simulink model "Main_model"  (R2021b)
settings: Solver=ode23t  StartTime=0.0  StopTime=sim_t_end  RelTol=1e-3
undefined symbols (not defined in the file): ambient_co2, ambient_pressure, ambient_rh, ambient_temp, battery, battery_heat_gen_scale, battery_mass, battery_thermal_mass, cab_air_v_dot, cabin_heater_cmd, cabin_heater_max_power, case_cold_plate_mass, case_cold_plate_thermal_mass, chiller_baffles_n, chiller_tube_length, chiller_tubes_n_rows, compressor_max_m_dot, compressor_ref_m_dot, condenser_air_min_flow_area, condenser_tube_width, const_current, coolant_channel_length, coolant_initial_T, coolant_m_dot, coolant_pipe_cross_sec_area, evaporator_air_cross_sec_area, evaporator_air_min_flow_area, evaporator_tube_width, motor_mc_heat_fraction, n_parallel, power_fraction_rear, ptc_heater_max_power, ptc_heater_thermal_mass, rad_air_v_dot, radiator_air_cross_sec_area, radiator_air_min_flow_area, radiator_tube_width, ref_m_dot, ref_pipe_dia, refrigerant_initial_void_fraction, refrigerant_pipe_cross_sec_area, T_bat_active_cool, T_bat_active_heat, T_bat_passive_cool, T_bat_passive_heat, T_battery_init, T_battery_nom, T_cabin_init, T_cabin_setpoint, T_dcdc_nom, T_DT_high, T_DT_passive_cool, T_DT_whr_active, T_front_gb_nom, T_front_mc_nom, T_front_motor_nom, T_rear_gb_nom, T_rear_mc_nom, T_rear_motor_nom, three_w_valve_max_open_area_factor ... (+3)
libraries: fl_lib x448, nesl_utility x328, SimscapeFluids_lib x134, slpidlib x15, ee_lib x9, simulink x8, LiBatteryElements_lib x4, SignalEditorBlockLib x1
(part 2 of 24)

== system Main_model/Compressor ==
  Absolute Reference (2P) : fl_lib/Two-Phase Fluid/Elements/Absolute Reference (2P)
      settings: SourceProductBaseCode=SS
  Absolute Reference (2P)1 : fl_lib/Two-Phase Fluid/Elements/Absolute Reference (2P)
      settings: SourceProductBaseCode=SS
  Constant1 : Constant  Value=1/.7-1
  Constant2 : Constant
  PS-Simulink Converter1 : nesl_utility/PS-Simulink Converter  PhysicalDomain=network_engine_domain  SubClassName=ps_output  LeftPortType=input  RightPortType=output  PseudoPeriodic=off  Frequencies=[]  Unit=MPa  AffineConversion=off
      settings: SourceProductBaseCode=PW,SS
  PS-Simulink Converter2 : nesl_utility/PS-Simulink Converter  PhysicalDomain=network_engine_domain  SubClassName=ps_output  LeftPortType=input  RightPortType=output  PseudoPeriodic=off  Frequencies=[]  Unit=MPa  AffineConversion=off
      settings: SourceProductBaseCode=PW,SS
  PS-Simulink Converter3 : nesl_utility/PS-Simulink Converter  PhysicalDomain=network_engine_domain  SubClassName=ps_output  LeftPortType=input  RightPortType=output  PseudoPeriodic=off  Frequencies=[]  Unit=K  AffineConversion=off
      settings: SourceProductBaseCode=PW,SS
  PS-Simulink Converter4 : nesl_utility/PS-Simulink Converter  PhysicalDomain=network_engine_domain  SubClassName=ps_output  LeftPortType=input  RightPortType=output  PseudoPeriodic=off  Frequencies=[]  Unit=K  AffineConversion=off
      settings: SourceProductBaseCode=PW,SS
  PS-Simulink Converter5 : nesl_utility/PS-Simulink Converter  PhysicalDomain=network_engine_domain  SubClassName=ps_output  LeftPortType=input  RightPortType=output  PseudoPeriodic=off  Frequencies=[]  Unit=1  AffineConversion=off
      settings: SourceProductBaseCode=PW,SS
  PS-Simulink Converter6 : nesl_utility/PS-Simulink Converter  PhysicalDomain=network_engine_domain  SubClassName=ps_output  LeftPortType=input  RightPortType=output  PseudoPeriodic=off  Frequencies=[]  Unit=1  AffineConversion=off
      settings: SourceProductBaseCode=PW,SS
  Pressure & Internal Energy Sensor (2P) : fl_lib/Two-Phase Fluid/Sensors/Pressure & Internal Energy Sensor (2P)
      settings: SourceProductBaseCode=SS  InternalSimscapePortConfiguration="{\"Bottom\":[],\"Left\":[{\"id\":\"A\",\"label\":\"A\",\"type\":\"foundation.two_phase_fluid.two_phase_fluid\"}],\"Right\":[{\"id\":\"B\",\"label\":\"B\",\"type\":\"foundation.two_phase_fluid.two_phase_fluid\"},{\"id\":\"P\",\"label\":\"P\",\"type\":\"output\"},{\"id\":\"U\",\"label\":\"U\",\"type\":\"output\"}],\"Top\":[]}"
  Pressure & Internal Energy Sensor (2P)1 : fl_lib/Two-Phase Fluid/Sensors/Pressure & Internal Energy Sensor (2P)
      settings: SourceProductBaseCode=SS  InternalSimscapePortConfiguration="{\"Bottom\":[],\"Left\":[{\"id\":\"A\",\"label\":\"A\",\"type\":\"foundation.two_phase_fluid.two_phase_fluid\"}],\"Right\":[{\"id\":\"B\",\"label\":\"B\",\"type\":\"foundation.two_phase_fluid.two_phase_fluid\"},{\"id\":\"P\",\"label\":\"P\",\"type\":\"output\"},{\"id\":\"U\",\"label\":\"U\",\"type\":\"output\"}],\"Top\":[]}"
  R1234yf Properties : SimscapeFluids_lib/Two-Phase Fluid/Utilities/Two-Phase Fluid Predefined Properties (2P)  fluid=fluids.two_phase_fluid.utilities.enum.Fluid.R1234yf  p_atm=ambient_pressure MPa  q_rev=0.01 Pa
      settings: SourceProductBaseCode=SH
  "Refrigerant Mass Flow Rate Controls " : Subsystem
  Scope : Scope
  Simulink-PS Converter1 : nesl_utility/Simulink-PS Converter  PhysicalDomain=network_engine_domain  SubClassName=ps_input  LeftPortType=input  RightPortType=output  PseudoPeriodic=off  Frequencies=[]  NoiseDistribution=none  NoiseParameters=[]  Unit=1  AffineConversion=off  FilteringAndDerivatives=provide  SimscapeFilterOrder=1  InputFilterTimeConstant=0.001  UdotUserProvided=0
      settings: SourceProductBaseCode=PW,SS
  Sum : Sum  Inputs=|++
  Thermodynamic Properties Sensor (2P) : fl_lib/Two-Phase Fluid/Sensors/Thermodynamic Properties Sensor (2P)
      settings: SourceProductBaseCode=SS  InternalSimscapePortConfiguration="{\"Bottom\":[],\"Left\":[{\"id\":\"A\",\"label\":\"A\",\"type\":\"foundation.two_phase_fluid.two_phase_fluid\"}],\"Right\":[{\"id\":\"T\",\"label\":\"T\",\"type\":\"output\"},{\"id\":\"H\",\"label\":\"h\",\"type\":\"output\"},{\"id\":\"V\",\"label\":\"v\",\"type\":\"output\"},{\"id\":\"S\",\"label\":\"s\",\"type\":\"output\"}],\"Top\":[]}"
  Thermodynamic Properties Sensor (2P)1 : fl_lib/Two-Phase Fluid/Sensors/Thermodynamic Properties Sensor (2P)
      settings: SourceProductBaseCode=SS  InternalSimscapePortConfiguration="{\"Bottom\":[],\"Left\":[{\"id\":\"A\",\"label\":\"A\",\"type\":\"foundation.two_phase_fluid.two_phase_fluid\"}],\"Right\":[{\"id\":\"T\",\"label\":\"T\",\"type\":\"output\"},{\"id\":\"H\",\"label\":\"h\",\"type\":\"output\"},{\"id\":\"V\",\"label\":\"v\",\"type\":\"output\"},{\"id\":\"S\",\"label\":\"s\",\"type\":\"output\"}],\"Top\":[]}"
  Transfer Fcn : TransferFcn  Denominator=[100 1]
  compressor : SimscapeComponentBlock  SourceFile=custom.self_controlled_mass_flow_source  ComponentPath=custom.self_controlled_mass_flow_source  ComponentVariants="[\"custom.self_controlled_mass_flow_source\"]"  ComponentVariantNames="[\"self_controlled_mass_flow_source\"]"  ClassName=self_controlled_mass_flow_source  SchemaVersion=1  power_spec=foundation.enum.power_spec.isentropic  area_A=refrigerant_pipe_cross_sec_area m^2  area_B=refrigerant_pipe_cross_sec_area m^2
      settings: CopyFcn=simscape.engine.sli.internal.componentblockcallback(gcbh,'COPY')  PreCopyFcn=simscape.engine.sli.internal.componentblockcallback(gcbh,'PRECOPY')  PreDeleteFcn=simscape.engine.sli.internal.componentblockcallback(gcbh,'PREDELETE')  InternalSimscapePortConfiguration="{\"Bottom\":[],\"Left\":[{\"id\":\"A\",\"label\":\"A\",\"type\":\"foundation.two_phase_fluid.two_phase_fluid\"},{\"id\":\"M\",\"label\":\"M\",\"type\":\"input\"},{\"id\":\"eff\",\"label\":\"eff\",\"type\":\"input\"}],\"Right\":[{\"id\":\"B\",\"label\":\"B\",\"type\":\"foundation.two_phase_fluid.two_phase_fluid\"}],\"Top\":[]}"
      mask Type: Controlled Mass Flow Rate Source (2P)
  heat loss : Subsystem
  Ref Out : PMIOPort  Side=Left
  Ref in : PMIOPort  Port=2  Side=Right
  tag scope: T_cond_comp_in=global, T_evap_comp_in=global, h_cond_comp_in=global, h_evap_comp_in=global, p_cond_comp_in=global, p_evap_comp_in=global
  wires:
  PS-Simulink Converter1/1 -> [p_evap_comp_in]
  PS-Simulink Converter2/1 -> [p_cond_comp_in]
  Sum/1 -> Scope/1, Simulink-PS Converter1/1
  Constant1/1 -> Transfer Fcn/1
  Constant2/1 -> Sum/2
  Transfer Fcn/1 -> Sum/1
  PS-Simulink Converter3/1 -> [T_evap_comp_in]
  PS-Simulink Converter5/1 -> [h_evap_comp_in]
  PS-Simulink Converter6/1 -> [h_cond_comp_in]
  PS-Simulink Converter4/1 -> [T_cond_comp_in]
  connections:
  PS-Simulink Converter1/LConn1 -- Pressure & Internal Energy Sensor (2P)/RConn2
  Pressure & Internal Energy Sensor (2P)/RConn1 -- Absolute Reference (2P)/LConn1
  Pressure & Internal Energy Sensor (2P)1/RConn1 -- Absolute Reference (2P)1/LConn1
  PS-Simulink Converter2/LConn1 -- Pressure & Internal Energy Sensor (2P)1/RConn2
  Pressure & Internal Energy Sensor (2P)1/LConn1 -- heat loss/LConn1 -- compressor/RConn1 -- Thermodynamic Properties Sensor (2P)1/LConn1
  heat loss/RConn1 -- Ref Out/RConn1
  "Refrigerant Mass Flow Rate Controls "/RConn1 -- compressor/LConn2
  compressor/LConn1 -- Pressure & Internal Energy Sensor (2P)/LConn1 -- R1234yf Properties/RConn1 -- Ref in/RConn1 -- Thermodynamic Properties Sensor (2P)/LConn1
  Simulink-PS Converter1/RConn1 -- compressor/LConn3
  Thermodynamic Properties Sensor (2P)/RConn2 -- PS-Simulink Converter5/LConn1
  PS-Simulink Converter3/LConn1 -- Thermodynamic Properties Sensor (2P)/RConn1
  Thermodynamic Properties Sensor (2P)1/RConn2 -- PS-Simulink Converter6/LConn1
  Thermodynamic Properties Sensor (2P)1/RConn1 -- PS-Simulink Converter4/LConn1

== system Main_model/Condenser ==
  Pump : Subsystem
  condenser : Subsystem
      settings: PortSchema="{\"entries\":[{\"content\":{\"sides\":[{\"content\":{\"connectorIds\":[]},\"type\":\"ConnectorPlacement.EquallySpacedRectSide\",\"uuid\":\"3be5e3bd-c423-4591-b0f7-380c1ba81e55\"},{\"content\":{\"connectorIds\":[],\"side\":\"RIGHT\"},\"type\":\"ConnectorPlacement.EquallySpacedRectSide\",\"uuid\":\"149d4538-0447-4c3c-bea8-6305fc9625c0\"},{\"content\":{\"connectorIds\":[\"LConn1\",\"LConn2\"],\"side\":\"TOP\"},\"type\":\"ConnectorPlacement.EquallySpacedRectSide\",\"uuid\":\"dd60c3f6-9393-4002-a01b-9d7c883b77f2\"}]},\"type\":\"ConnectorPlacement.EquallySpacedConnector\",\"uuid\":\"8455fa94-fdd0-4f54-8085-fe1f60725002\"}],\"packageUris\":[\"http://schema.mathworks.com/mf0/Connector/R2020b\"],\"version\":\"1.0\"}"
  condenser1 : Subsystem  Commented=on
  LCC O : PMIOPort  Side=Right
  LCC In : PMIOPort  Port=2  Side=Right
  Ch O : PMIOPort  Port=3  Side=Right
  Ch I : PMIOPort  Port=4  Side=Right
  connections:
  LCC O/RConn1 -- condenser/LConn2 -- Ch O/RConn1
  LCC In/RConn1 -- Pump/LConn1 -- Ch I/RConn1
  condenser/LConn1 -- Pump/RConn1

== system Main_model/DT, Bat Temp tracking and Radiator Fan speed ==
  Constant : Constant  Value=T_battery_nom
  Constant1 : Constant  Value=T_dcdc_nom
  Constant10 : Constant  Value=ambient_temp
  Constant2 : Constant  Value=T_front_gb_nom
  Constant3 : Constant  Value=T_rear_gb_nom
  Constant4 : Constant  Value=T_front_mc_nom
  Constant5 : Constant  Value=T_rear_mc_nom
  Constant6 : Constant  Value=T_front_motor_nom
  Constant7 : Constant  Value=T_rear_motor_nom
  Constant9 : Constant  Value=.5
  Data Type Conversion2 : DataTypeConversion
  Gain : Gain  Gain=1/8*1/2
  Min : MinMax  Inputs=6
  Min1 : MinMax  Function=max  Inputs=6
  Min2 : MinMax  Inputs=2
  Mux2 : Mux  Inputs=9
  Relational Operator{,1..7} (8 alike) : RelationalOperator  Operator=>  OutDataTypeStr=boolean  RndMeth=Simplest
  Scope : Scope  NumInputPorts=2
  Sum : Sum  Inputs=|++++++++
  Sum1 : Sum  Inputs=|++
  Transfer Fcn1 : TransferFcn  Denominator=[1 1]
  tag scope: T_DT=global, T_DT_max=global, T_DT_min=global, T_gb_min=global, cmd_fan=global
  wires:
  [T_dcdc] -> Relational Operator1/1, Mux2/2  "dc dc"
  Relational Operator4/1 -> Sum/5
  Mux2/1 -> Scope/1, [T_DT]
  [T_front_mc] -> Relational Operator4/1, Min/3, Min1/3, Mux2/5  "front mc"
  [T_rear_gb] -> Min2/1, Min/2, Min1/2, Mux2/4, Relational Operator3/1  "rear gb"
  Sum/1 -> Data Type Conversion2/1
  Relational Operator5/1 -> Sum/6
  [T_front_gb] -> Relational Operator2/1, Min2/2, Min/1, Min1/1, Mux2/3  "front gb"
  Relational Operator/1 -> Sum/1
  Constant7/1 -> Relational Operator7/2
  Constant3/1 -> Relational Operator3/2
  [T_battery] -> Relational Operator/1, Mux2/1  "battery"
  Relational Operator1/1 -> Sum/2
  Relational Operator3/1 -> Sum/4
  Relational Operator6/1 -> Sum/7
  Relational Operator7/1 -> Sum/8
  Relational Operator2/1 -> Sum/3
  Constant/1 -> Relational Operator/2
  [T_rear_motor] -> Relational Operator7/1, Min/6, Min1/6, Mux2/8  "rear motor"
  [T_front_motor] -> Relational Operator6/1, Min/5, Min1/5, Mux2/7  "front motor"
  [T_rear_mc] -> Min/4, Min1/4, Mux2/6, Relational Operator5/1  "rear mc"
  Constant4/1 -> Relational Operator4/2
  Constant5/1 -> Relational Operator5/2
  Constant2/1 -> Relational Operator2/2
  Constant6/1 -> Relational Operator6/2
  Constant1/1 -> Relational Operator1/2
  Data Type Conversion2/1 -> Gain/1
  Gain/1 -> Sum1/1
  Constant9/1 -> Sum1/2
  Sum1/1 -> Transfer Fcn1/1
  Transfer Fcn1/1 -> Scope/2, [cmd_fan]  "cmd fan speed"
  Constant10/1 -> Mux2/9  "ambient"
  Min/1 -> [T_DT_min]
  Min1/1 -> [T_DT_max]
  Min2/1 -> [T_gb_min]

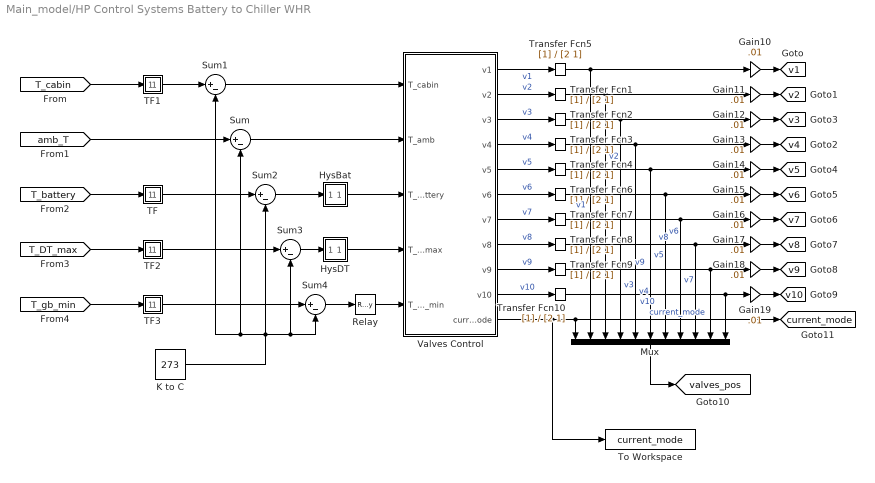
== system Main_model/HP Control Systems Battery to Chiller WHR  ==
  Gain{10..19} (10 alike) : Gain  Gain=.01
  HysBat : Subsystem
  HysDT : Subsystem
  K to C : Constant  Value=273
  Mux : Mux  Inputs=11
  Relay : Relay  OnSwitchValue=T_DT_whr_active  OffSwitchValue=T_DT_whr_active-5  OnOutputValue=T_DT_whr_active*1.1  OffOutputValue=T_DT_whr_active*.9
  Sum{,1..4} (5 alike) : Sum  Inputs=|+-
  TF : Subsystem
  TF1 : Subsystem
  TF2 : Subsystem
  TF3 : Subsystem
  To Workspace : ToWorkspace  VariableName=current_mode  SaveFormat=Timeseries  SampleTime=-1
  Transfer Fcn{1..10} (10 alike) : TransferFcn  Denominator=[2 1]
  Valves Control : MATLAB Function  TreatAsAtomicUnit=on
  tag scope: current_mode=global, v10=global, v1=global, v2=global, v3=global, v4=global, v5=global, v6=global, v7=global, v8=global, v9=global, valves_pos=global
  wires:
  Relay/1 -> Valves Control/5(T_DT_min)
  HysDT/1(Out1) -> Valves Control/4(T_DT_max)
  TF/1(Out1) -> Sum2/1
  TF2/1(Out1) -> Sum3/1
  TF3/1(Out1) -> Sum4/1
  TF1/1(Out1) -> Sum1/1
  [T_DT_max] -> TF2/1(In1)
  [T_cabin] -> TF1/1(In1)
  [T_battery] -> TF/1(In1)
  [T_gb_min] -> TF3/1(In1)
  Valves Control/2(v2) -> Transfer Fcn1/1  "v2"
  K to C/1 -> Sum1/2, Sum/2, Sum2/2, Sum3/2, Sum4/2
  Sum2/1 -> HysBat/1(In1)
  Sum/1 -> Valves Control/2(T_amb)
  Valves Control/5(v5) -> Transfer Fcn4/1  "v5"
  Valves Control/10(v10) -> Transfer Fcn10/1  "v10"
  Valves Control/4(v4) -> Transfer Fcn3/1  "v4"
  Gain18/1 -> [v9]
  Valves Control/6(v6) -> Transfer Fcn6/1  "v6"
  Transfer Fcn3/1 -> Gain13/1, Mux/5  "v4"
  Transfer Fcn10/1 -> Mux/11, Gain19/1  "v10"
  Transfer Fcn6/1 -> Gain15/1, Mux/7  "v6"
  Gain10/1 -> [v1]
  Transfer Fcn8/1 -> Mux/9, Gain17/1  "v8"
  Valves Control/3(v3) -> Transfer Fcn2/1  "v3"
  Transfer Fcn2/1 -> Mux/4, Gain12/1  "v3"
  Gain11/1 -> [v2]
  Transfer Fcn9/1 -> Mux/10, Gain18/1  "v9"
  Sum4/1 -> Relay/1
  Gain19/1 -> [v10]
  Transfer Fcn1/1 -> Mux/3, Gain11/1  "v2"
  Gain12/1 -> [v3]
  Gain14/1 -> [v5]
  Valves Control/9(v9) -> Transfer Fcn9/1  "v9"
  Gain16/1 -> [v7]
  HysBat/1(Out1) -> Valves Control/3(T_battery)
  Gain17/1 -> [v8]
  Valves Control/11(current_mode) -> To Workspace/1, Mux/1, [current_mode]  "current_mode"
  Gain13/1 -> [v4]
  Transfer Fcn4/1 -> Gain14/1, Mux/6  "v5"
  Sum1/1 -> Valves Control/1(T_cabin)
  Valves Control/7(v7) -> Transfer Fcn7/1  "v7"
  Valves Control/8(v8) -> Transfer Fcn8/1  "v8"
  Transfer Fcn5/1 -> Gain10/1, Mux/2  "v1"
  Gain15/1 -> [v6]
  Valves Control/1(v1) -> Transfer Fcn5/1  "v1"
  Mux/1 -> [valves_pos]
  [amb_T] -> Sum/1
  Transfer Fcn7/1 -> Mux/8, Gain16/1  "v7"
  Sum3/1 -> HysDT/1(In1)

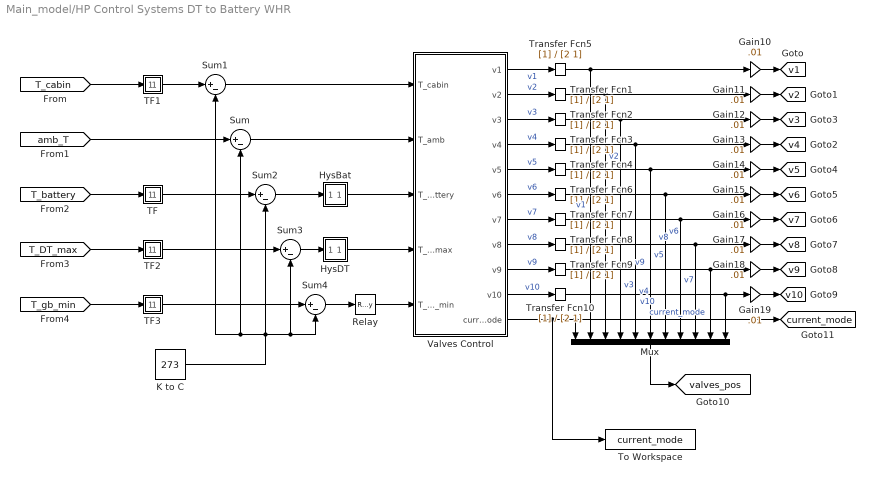
== system Main_model/HP Control Systems DT to Battery WHR  ==
  Gain{10..19} (10 alike) : Gain  Gain=.01
  HysBat : Subsystem
  HysDT : Subsystem
  K to C : Constant  Value=273
  Mux : Mux  Inputs=11
  Relay : Relay  OnSwitchValue=T_DT_whr_active  OffSwitchValue=T_DT_whr_active-5  OnOutputValue=T_DT_whr_active*1.1  OffOutputValue=T_DT_whr_active*.9
  Sum{,1..4} (5 alike) : Sum  Inputs=|+-
  TF : Subsystem
  TF1 : Subsystem
  TF2 : Subsystem
  TF3 : Subsystem
  To Workspace : ToWorkspace  VariableName=current_mode  SaveFormat=Timeseries  SampleTime=-1
  Transfer Fcn{1..10} (10 alike) : TransferFcn  Denominator=[2 1]
  Valves Control : MATLAB Function  TreatAsAtomicUnit=on
  tag scope: current_mode=global, v10=global, v1=global, v2=global, v3=global, v4=global, v5=global, v6=global, v7=global, v8=global, v9=global, valves_pos=global
  wires:
  Relay/1 -> Valves Control/5(T_DT_min)
  HysDT/1(Out1) -> Valves Control/4(T_DT_max)
  TF/1(Out1) -> Sum2/1
  TF2/1(Out1) -> Sum3/1
  TF3/1(Out1) -> Sum4/1
  TF1/1(Out1) -> Sum1/1
  [T_DT_max] -> TF2/1(In1)
  [T_cabin] -> TF1/1(In1)
  [T_battery] -> TF/1(In1)
  [T_gb_min] -> TF3/1(In1)
  Valves Control/2(v2) -> Transfer Fcn1/1  "v2"
  K to C/1 -> Sum1/2, Sum/2, Sum2/2, Sum3/2, Sum4/2
  Sum2/1 -> HysBat/1(In1)
  Sum/1 -> Valves Control/2(T_amb)
  Valves Control/5(v5) -> Transfer Fcn4/1  "v5"
  Valves Control/10(v10) -> Transfer Fcn10/1  "v10"
  Valves Control/4(v4) -> Transfer Fcn3/1  "v4"
  Gain18/1 -> [v9]
  Valves Control/6(v6) -> Transfer Fcn6/1  "v6"
  Transfer Fcn3/1 -> Gain13/1, Mux/5  "v4"
  Transfer Fcn10/1 -> Mux/11, Gain19/1  "v10"
  Transfer Fcn6/1 -> Gain15/1, Mux/7  "v6"
  Gain10/1 -> [v1]
  Transfer Fcn8/1 -> Mux/9, Gain17/1  "v8"
  Valves Control/3(v3) -> Transfer Fcn2/1  "v3"
  Transfer Fcn2/1 -> Mux/4, Gain12/1  "v3"
  Gain11/1 -> [v2]
  Transfer Fcn9/1 -> Mux/10, Gain18/1  "v9"
  Sum4/1 -> Relay/1
  Gain19/1 -> [v10]
  Transfer Fcn1/1 -> Mux/3, Gain11/1  "v2"
  Gain12/1 -> [v3]
  Gain14/1 -> [v5]
  Valves Control/9(v9) -> Transfer Fcn9/1  "v9"
  Gain16/1 -> [v7]
  HysBat/1(Out1) -> Valves Control/3(T_battery)
  Gain17/1 -> [v8]
  Valves Control/11(current_mode) -> To Workspace/1, Mux/1, [current_mode]  "current_mode"
  Gain13/1 -> [v4]
  Transfer Fcn4/1 -> Gain14/1, Mux/6  "v5"
  Sum1/1 -> Valves Control/1(T_cabin)
  Valves Control/7(v7) -> Transfer Fcn7/1  "v7"
  Valves Control/8(v8) -> Transfer Fcn8/1  "v8"
  Transfer Fcn5/1 -> Gain10/1, Mux/2  "v1"
  Gain15/1 -> [v6]
  Valves Control/1(v1) -> Transfer Fcn5/1  "v1"
  Mux/1 -> [valves_pos]
  [amb_T] -> Sum/1
  Transfer Fcn7/1 -> Mux/8, Gain16/1  "v7"
  Sum3/1 -> HysDT/1(In1)

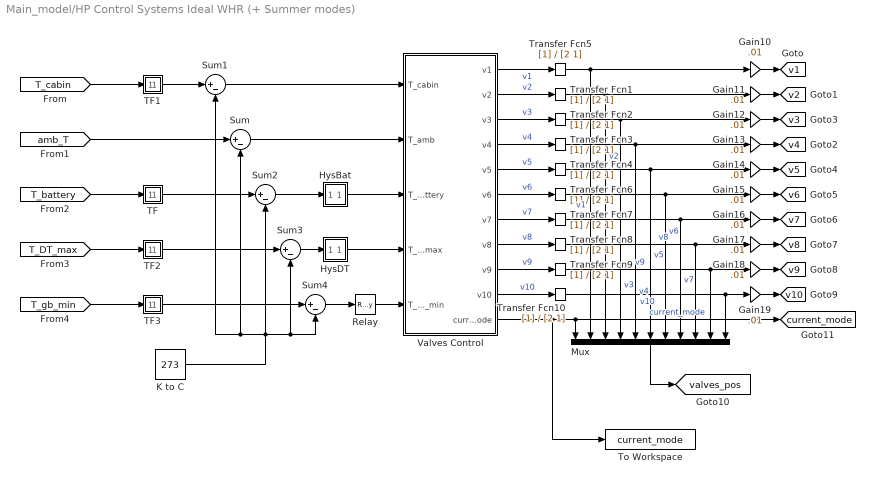
== system Main_model/HP Control Systems Ideal WHR (+ Summer modes)  ==
  Gain{10..19} (10 alike) : Gain  Gain=.01
  HysBat : Subsystem
  HysDT : Subsystem
  K to C : Constant  Value=273
  Mux : Mux  Inputs=11
  Relay : Relay  OnSwitchValue=T_DT_whr_active  OffSwitchValue=T_DT_whr_active-5  OnOutputValue=T_DT_whr_active*1.1  OffOutputValue=T_DT_whr_active*.9
  Sum{,1..4} (5 alike) : Sum  Inputs=|+-
  TF : Subsystem
  TF1 : Subsystem
  TF2 : Subsystem
  TF3 : Subsystem
  To Workspace : ToWorkspace  VariableName=current_mode  SaveFormat=Timeseries  SampleTime=-1
  Transfer Fcn{1..10} (10 alike) : TransferFcn  Denominator=[2 1]
  Valves Control : MATLAB Function  TreatAsAtomicUnit=on
  tag scope: current_mode=global, v10=global, v1=global, v2=global, v3=global, v4=global, v5=global, v6=global, v7=global, v8=global, v9=global, valves_pos=global
  wires:
  Valves Control/4(v4) -> Transfer Fcn3/1  "v4"
  Valves Control/3(v3) -> Transfer Fcn2/1  "v3"
  Valves Control/2(v2) -> Transfer Fcn1/1  "v2"
  Valves Control/1(v1) -> Transfer Fcn5/1  "v1"
  Valves Control/5(v5) -> Transfer Fcn4/1  "v5"
  Valves Control/6(v6) -> Transfer Fcn6/1  "v6"
  Valves Control/8(v8) -> Transfer Fcn8/1  "v8"
  Valves Control/9(v9) -> Transfer Fcn9/1  "v9"
  Valves Control/10(v10) -> Transfer Fcn10/1  "v10"
  Mux/1 -> [valves_pos]
  [amb_T] -> Sum/1
  Sum1/1 -> Valves Control/1(T_cabin)
  Sum/1 -> Valves Control/2(T_amb)
  Sum2/1 -> HysBat/1(In1)
  K to C/1 -> Sum1/2, Sum/2, Sum2/2, Sum3/2, Sum4/2
  Valves Control/11(current_mode) -> To Workspace/1, Mux/1, [current_mode]  "current_mode"
  [T_cabin] -> TF1/1(In1)
  [T_battery] -> TF/1(In1)
  Transfer Fcn5/1 -> Gain10/1, Mux/2  "v1"
  Transfer Fcn1/1 -> Mux/3, Gain11/1  "v2"
  Transfer Fcn2/1 -> Mux/4, Gain12/1  "v3"
  Transfer Fcn3/1 -> Gain13/1, Mux/5  "v4"
  Transfer Fcn4/1 -> Gain14/1, Mux/6  "v5"
  Transfer Fcn6/1 -> Gain15/1, Mux/7  "v6"
  Transfer Fcn7/1 -> Mux/8, Gain16/1  "v7"
  Transfer Fcn8/1 -> Mux/9, Gain17/1  "v8"
  Transfer Fcn9/1 -> Mux/10, Gain18/1  "v9"
  Transfer Fcn10/1 -> Mux/11, Gain19/1  "v10"
  Gain10/1 -> [v1]
  Gain11/1 -> [v2]
  Gain12/1 -> [v3]
  Gain13/1 -> [v4]
  Gain14/1 -> [v5]
  Gain15/1 -> [v6]
  Gain16/1 -> [v7]
  Gain17/1 -> [v8]
  Gain18/1 -> [v9]
  Gain19/1 -> [v10]
  Valves Control/7(v7) -> Transfer Fcn7/1  "v7"
  TF1/1(Out1) -> Sum1/1
  TF/1(Out1) -> Sum2/1
  [T_DT_max] -> TF2/1(In1)
  [T_gb_min] -> TF3/1(In1)
  Sum4/1 -> Relay/1
  Sum3/1 -> HysDT/1(In1)
  TF2/1(Out1) -> Sum3/1
  TF3/1(Out1) -> Sum4/1
  HysDT/1(Out1) -> Valves Control/4(T_DT_max)
  Relay/1 -> Valves Control/5(T_DT_min)
  HysBat/1(Out1) -> Valves Control/3(T_battery)

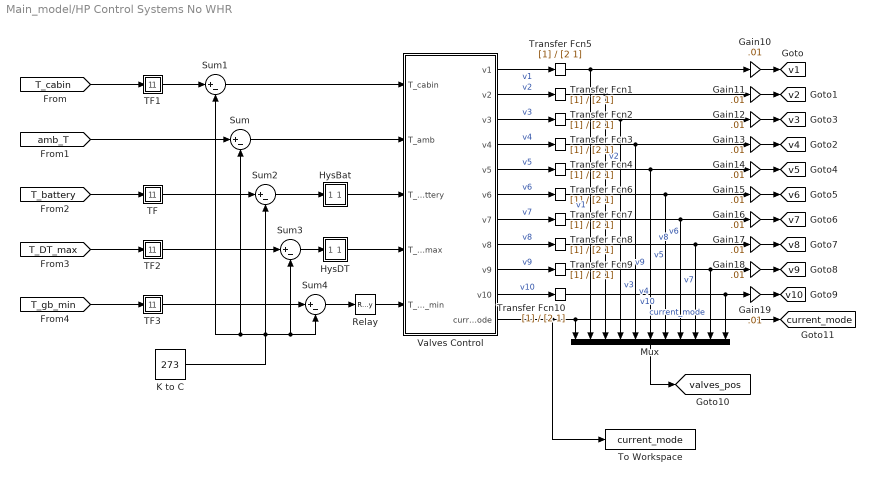
== system Main_model/HP Control Systems No WHR ==
  Gain{10..19} (10 alike) : Gain  Gain=.01
  HysBat : Subsystem
  HysDT : Subsystem
  K to C : Constant  Value=273
  Mux : Mux  Inputs=11
  Relay : Relay  OnSwitchValue=T_DT_whr_active  OffSwitchValue=T_DT_whr_active-5  OnOutputValue=T_DT_whr_active*1.1  OffOutputValue=T_DT_whr_active*.9
  Sum{,1..4} (5 alike) : Sum  Inputs=|+-
  TF : Subsystem
  TF1 : Subsystem
  TF2 : Subsystem
  TF3 : Subsystem
  To Workspace : ToWorkspace  VariableName=current_mode  SaveFormat=Timeseries  SampleTime=-1
  Transfer Fcn{1..10} (10 alike) : TransferFcn  Denominator=[2 1]
  Valves Control : MATLAB Function  TreatAsAtomicUnit=on
  tag scope: current_mode=global, v10=global, v1=global, v2=global, v3=global, v4=global, v5=global, v6=global, v7=global, v8=global, v9=global, valves_pos=global
  wires:
  Relay/1 -> Valves Control/5(T_DT_min)
  HysDT/1(Out1) -> Valves Control/4(T_DT_max)
  TF/1(Out1) -> Sum2/1
  TF2/1(Out1) -> Sum3/1
  TF3/1(Out1) -> Sum4/1
  TF1/1(Out1) -> Sum1/1
  [T_DT_max] -> TF2/1(In1)
  [T_cabin] -> TF1/1(In1)
  [T_battery] -> TF/1(In1)
  [T_gb_min] -> TF3/1(In1)
  Valves Control/2(v2) -> Transfer Fcn1/1  "v2"
  K to C/1 -> Sum1/2, Sum/2, Sum2/2, Sum3/2, Sum4/2
  Sum2/1 -> HysBat/1(In1)
  Sum/1 -> Valves Control/2(T_amb)
  Valves Control/5(v5) -> Transfer Fcn4/1  "v5"
  Valves Control/10(v10) -> Transfer Fcn10/1  "v10"
  Valves Control/4(v4) -> Transfer Fcn3/1  "v4"
  Gain18/1 -> [v9]
  Valves Control/6(v6) -> Transfer Fcn6/1  "v6"
  Transfer Fcn3/1 -> Gain13/1, Mux/5  "v4"
  Transfer Fcn10/1 -> Mux/11, Gain19/1  "v10"
  Transfer Fcn6/1 -> Gain15/1, Mux/7  "v6"
  Gain10/1 -> [v1]
  Transfer Fcn8/1 -> Mux/9, Gain17/1  "v8"
  Valves Control/3(v3) -> Transfer Fcn2/1  "v3"
  Transfer Fcn2/1 -> Mux/4, Gain12/1  "v3"
  Gain11/1 -> [v2]
  Transfer Fcn9/1 -> Mux/10, Gain18/1  "v9"
  Sum4/1 -> Relay/1
  Gain19/1 -> [v10]
  Transfer Fcn1/1 -> Mux/3, Gain11/1  "v2"
  Gain12/1 -> [v3]
  Gain14/1 -> [v5]
  Valves Control/9(v9) -> Transfer Fcn9/1  "v9"
  Gain16/1 -> [v7]
  HysBat/1(Out1) -> Valves Control/3(T_battery)
  Gain17/1 -> [v8]
  Valves Control/11(current_mode) -> To Workspace/1, Mux/1, [current_mode]  "current_mode"
  Gain13/1 -> [v4]
  Transfer Fcn4/1 -> Gain14/1, Mux/6  "v5"
  Sum1/1 -> Valves Control/1(T_cabin)
  Valves Control/7(v7) -> Transfer Fcn7/1  "v7"
  Valves Control/8(v8) -> Transfer Fcn8/1  "v8"
  Transfer Fcn5/1 -> Gain10/1, Mux/2  "v1"
  Gain15/1 -> [v6]
  Valves Control/1(v1) -> Transfer Fcn5/1  "v1"
  Mux/1 -> [valves_pos]
  [amb_T] -> Sum/1
  Transfer Fcn7/1 -> Mux/8, Gain16/1  "v7"
  Sum3/1 -> HysDT/1(In1)

== system Main_model/HP Control Systems Only DT to Chiller WHR ==
  Gain{10..19} (10 alike) : Gain  Gain=.01
  HysBat : Subsystem
  HysDT : Subsystem
  K to C : Constant  Value=273
  Mux : Mux  Inputs=11
  Relay : Relay  OnSwitchValue=T_DT_whr_active  OffSwitchValue=T_DT_whr_active-5  OnOutputValue=T_DT_whr_active*1.1  OffOutputValue=T_DT_whr_active*.9
  Sum{,1..4} (5 alike) : Sum  Inputs=|+-
  TF : Subsystem
  TF1 : Subsystem
  TF2 : Subsystem
  TF3 : Subsystem
  To Workspace : ToWorkspace  VariableName=current_mode  SaveFormat=Timeseries  SampleTime=-1
  Transfer Fcn{1..10} (10 alike) : TransferFcn  Denominator=[2 1]
  Valves Control : MATLAB Function  TreatAsAtomicUnit=on
  tag scope: current_mode=global, v10=global, v1=global, v2=global, v3=global, v4=global, v5=global, v6=global, v7=global, v8=global, v9=global, valves_pos=global
  wires:
  Relay/1 -> Valves Control/5(T_DT_min)
  HysDT/1(Out1) -> Valves Control/4(T_DT_max)
  TF/1(Out1) -> Sum2/1
  TF2/1(Out1) -> Sum3/1
  TF3/1(Out1) -> Sum4/1
  TF1/1(Out1) -> Sum1/1
  [T_DT_max] -> TF2/1(In1)
  [T_cabin] -> TF1/1(In1)
  [T_battery] -> TF/1(In1)
  [T_gb_min] -> TF3/1(In1)
  Valves Control/2(v2) -> Transfer Fcn1/1  "v2"
  K to C/1 -> Sum1/2, Sum/2, Sum2/2, Sum3/2, Sum4/2
  Sum2/1 -> HysBat/1(In1)
  Sum/1 -> Valves Control/2(T_amb)
  Valves Control/5(v5) -> Transfer Fcn4/1  "v5"
  Valves Control/10(v10) -> Transfer Fcn10/1  "v10"
  Valves Control/4(v4) -> Transfer Fcn3/1  "v4"
  Gain18/1 -> [v9]
  Valves Control/6(v6) -> Transfer Fcn6/1  "v6"
  Transfer Fcn3/1 -> Gain13/1, Mux/5  "v4"
  Transfer Fcn10/1 -> Mux/11, Gain19/1  "v10"
  Transfer Fcn6/1 -> Gain15/1, Mux/7  "v6"
  Gain10/1 -> [v1]
  Transfer Fcn8/1 -> Mux/9, Gain17/1  "v8"
  Valves Control/3(v3) -> Transfer Fcn2/1  "v3"
  Transfer Fcn2/1 -> Mux/4, Gain12/1  "v3"
  Gain11/1 -> [v2]
  Transfer Fcn9/1 -> Mux/10, Gain18/1  "v9"
  Sum4/1 -> Relay/1
  Gain19/1 -> [v10]
  Transfer Fcn1/1 -> Mux/3, Gain11/1  "v2"
  Gain12/1 -> [v3]
  Gain14/1 -> [v5]
  Valves Control/9(v9) -> Transfer Fcn9/1  "v9"
  Gain16/1 -> [v7]
  HysBat/1(Out1) -> Valves Control/3(T_battery)
  Gain17/1 -> [v8]
  Valves Control/11(current_mode) -> To Workspace/1, Mux/1, [current_mode]  "current_mode"
  Gain13/1 -> [v4]
  Transfer Fcn4/1 -> Gain14/1, Mux/6  "v5"
  Sum1/1 -> Valves Control/1(T_cabin)
  Valves Control/7(v7) -> Transfer Fcn7/1  "v7"
  Valves Control/8(v8) -> Transfer Fcn8/1  "v8"
  Transfer Fcn5/1 -> Gain10/1, Mux/2  "v1"
  Gain15/1 -> [v6]
  Valves Control/1(v1) -> Transfer Fcn5/1  "v1"
  Mux/1 -> [valves_pos]
  [amb_T] -> Sum/1
  Transfer Fcn7/1 -> Mux/8, Gain16/1  "v7"
  Sum3/1 -> HysDT/1(In1)

== system Main_model/HVAC cycles ==
  note: Direct Configuration
  note: Compressor Control (Keep Uncommented for both configs)
  note: Cabin Direct Cooling Heating
  note: HVAC1
  note: HVAC4
  note: Cabin
  note: Different Direct-Indirect Configs (Uncomment only one)
      | Comment ' Heat Loss Signals from Autonomie', 'DT, Bat Temp tracking and Radiator Fan speed', GIL framework and WHR control algos.
      | Use the following initialisation file - 'cabin_conditioning_parameters_initialisation.m'
  note: Ind irect Configuration
  note: Save results of Direct configuration as out1 and that of indirect as out4 for post-processing and analysis by the scripts.
  4 Way Valve (2P)2 : Subsystem  Commented=on
  4 Way Valve (2P)3 : Subsystem
  Compressor On-Off : Subsystem
  LCC4 : Subsystem  Commented=on
  TXV1 : Subsystem
  TXV4 : Subsystem  Commented=on
  cabin HX4 : Subsystem  Commented=on
      settings: PortSchema="{\"entries\":[{\"content\":{\"sides\":[{\"content\":{\"connectorIds\":[]},\"type\":\"ConnectorPlacement.EquallySpacedRectSide\",\"uuid\":\"71822b2c-9ca3-4cc9-92d1-ecf472f04bd4\"},{\"content\":{\"connectorIds\":[],\"side\":\"RIGHT\"},\"type\":\"ConnectorPlacement.EquallySpacedRectSide\",\"uuid\":\"e0df667d-86dd-460a-bd26-f563eb1ee1db\"},{\"content\":{\"connectorIds\":[\"LConn1\",\"LConn2\"],\"side\":\"TOP\"},\"type\":\"ConnectorPlacement.EquallySpacedRectSide\",\"uuid\":\"56daad42-8202-443d-af27-a6baa0bd3366\"},{\"content\":{\"connectorIds\":[\"RConn1\",\"RConn2\"],\"side\":\"BOTTOM\"},\"type\":\"ConnectorPlacement.EquallySpacedRectSide\",\"uuid\":\"4778d153-f81a-4fb0-9678-a5e1ef62924d\"}]},\"type\":\"ConnectorPlacement.EquallySpacedConnector\",\"uuid\":\"488efe04-0e39-4e1b-8b30-4bca48b36ba3\"}],\"packageUris\":[\"http://schema.mathworks.com/mf0/Connector/R2020b\"],\"version\":\"1.0\"}"
  cabin evap1 : Subsystem
  cabin1 : Subsystem
  cabin4 : Subsystem  Commented=on
  chiller4 : Subsystem  Commented=on
  compressor1 : Subsystem
  compressor4 : Subsystem  Commented=on
  condenser1 : Subsystem
  pump4_1 : Subsystem  Commented=on
  pump4_2 : Subsystem  Commented=on
  radiator4 : Subsystem  Commented=on
  connections:
  4 Way Valve (2P)3/RConn2 -- compressor1/RConn2 -- TXV1/LConn3
  4 Way Valve (2P)2/RConn2 -- TXV4/LConn3 -- compressor4/RConn2
  cabin1/RConn2 -- cabin evap1/LConn4
  cabin1/RConn1 -- cabin evap1/LConn3
  TXV1/LConn1 -- cabin evap1/LConn1
  cabin4/RConn2 -- cabin HX4/LConn2
  TXV1/LConn2 -- condenser1/LConn2
  cabin4/RConn1 -- cabin HX4/LConn1
  radiator4/LConn1 -- LCC4/LConn1
  compressor1/RConn1 -- 4 Way Valve (2P)3/LConn1
  chiller4/RConn2 -- 4 Way Valve (2P)2/LConn2
  LCC4/RConn1 -- 4 Way Valve (2P)2/RConn1
  LCC4/RConn2 -- TXV4/LConn2
  chiller4/RConn1 -- TXV4/LConn1
  cabin evap1/LConn2 -- 4 Way Valve (2P)3/LConn2
  pump4_2/RConn1 -- cabin HX4/RConn2
  compressor4/RConn1 -- 4 Way Valve (2P)2/LConn1
  condenser1/LConn1 -- 4 Way Valve (2P)3/RConn1
  cabin HX4/RConn1 -- chiller4/LConn2
  chiller4/LConn1 -- pump4_2/LConn1
  pump4_1/LConn1 -- radiator4/LConn2
  LCC4/LConn2 -- pump4_1/RConn1

== system Main_model/Individual Component Analysis ==
  note: Individual Component Analysis Setup for Different Components (Uncomment only one)
      |
      | Comment GIL, WHR control algos, 'Autonomie Heat Generation Data' and 'DT, Bat Temp tracking and Radiator Fan speed' blocks
  Reservoir (2P)1 : fl_lib/Two-Phase Fluid/Elements/Reservoir (2P)  Commented=on  pressure_spec=foundation.enum.ReservoirPressureSpec2P.Specified  reservoir_pressure=ref_P MPa  reservoir_condensing_temperature=ref_T_in K  reservoir_evaporating_temperature=373.15 K  energy_spec=foundation.enum.ReservoirEnergySpec2P.Temperature  reservoir_temperature=ref_T_in K  reservoir_quality=0.5  reservoir_void_fraction=0.5  reservoir_enthalpy=1500 kJ/kg  reservoir_internal_energy=1500 kJ/kg  reservoir_subcooling=5 deltaK  reservoir_superheating=5 deltaK  area_A=refrigerant_pipe_cross_sec_area m^2
      settings: SourceProductBaseCode=SS
  Reservoir (2P)2 : fl_lib/Two-Phase Fluid/Elements/Reservoir (2P)  Commented=on  pressure_spec=foundation.enum.ReservoirPressureSpec2P.Specified  reservoir_pressure=ref_P MPa  reservoir_condensing_temperature=ref_T_in K  reservoir_evaporating_temperature=373.15 K  energy_spec=foundation.enum.ReservoirEnergySpec2P.Temperature  reservoir_temperature=ref_T_in K  reservoir_quality=0.5  reservoir_void_fraction=0.5  reservoir_enthalpy=1500 kJ/kg  reservoir_internal_energy=1500 kJ/kg  reservoir_subcooling=5 deltaK  reservoir_superheating=5 deltaK  area_A=refrigerant_pipe_cross_sec_area m^2
      settings: SourceProductBaseCode=SS
  Reservoir (TL){1,4,7,9} (4 alike) : fl_lib/Thermal Liquid/Elements/Reservoir (TL)  Commented=on  pressure_spec=foundation.enum.pressure_spec.atmospheric  reservoir_pressure=0.101325 MPa  reservoir_temperature=ambient_temp K  area=coolant_pipe_cross_sec_area m^2
      settings: SourceProductBaseCode=SS
  Reservoir (TL){2,5,8,10} (4 alike) : fl_lib/Thermal Liquid/Elements/Reservoir (TL)  Commented=on  pressure_spec=foundation.enum.pressure_spec.atmospheric  reservoir_pressure=0.101325 MPa  reservoir_temperature=coolant_T_in K  area=coolant_pipe_cross_sec_area m^2
      settings: SourceProductBaseCode=SS
  cabin_hx : Subsystem  Commented=on
  chiller : Subsystem  Commented=on
  heat_gen_comp : Subsystem  Commented=on
  pump : Subsystem  Commented=on
  pump1 : Subsystem  Commented=on
  pump2 : Subsystem  Commented=on
  pump5 : Subsystem  Commented=on
  pump6 : Subsystem  Commented=on
  radiator : Subsystem  Commented=on
  connections:
  Reservoir (TL)5/LConn1 -- pump/RConn1
  Reservoir (TL)2/LConn1 -- pump1/RConn1
  pump1/LConn1 -- chiller/LConn1
  Reservoir (2P)2/LConn1 -- chiller/LConn2
  Reservoir (TL)1/LConn1 -- chiller/RConn1
  Reservoir (2P)1/LConn1 -- pump2/RConn1
  pump/LConn1 -- radiator/LConn1
  Reservoir (TL)4/LConn1 -- radiator/RConn1
  pump2/LConn1 -- chiller/RConn2
  Reservoir (TL)7/LConn1 -- cabin_hx/RConn1
  pump5/LConn1 -- cabin_hx/LConn1
  Reservoir (TL)8/LConn1 -- pump5/RConn1
  Reservoir (TL)10/LConn1 -- pump6/RConn1
  pump6/LConn1 -- heat_gen_comp/LConn1
  Reservoir (TL)9/LConn1 -- heat_gen_comp/RConn1

== system Main_model/LCC ==
  note: Keep PTC Heater commneted for HP configs. analysis. Follow the steps mentioned in the script- paper_1_pager_heat_flow_ptc.m for PTC analysis
  Absolute Reference (TL) : fl_lib/Thermal Liquid/Elements/Absolute Reference (TL)
      settings: SourceProductBaseCode=SS
  LCC : Subsystem
  PS-Simulink Converter : nesl_utility/PS-Simulink Converter  PhysicalDomain=network_engine_domain  SubClassName=ps_output  LeftPortType=input  RightPortType=output  PseudoPeriodic=off  Frequencies=[]  Unit=inherit  AffineConversion=off
      settings: SourceProductBaseCode=PW,SS
  PTC Heater : Subsystem  Commented=on
  Pressure & Temperature Sensor (TL) : fl_lib/Thermal Liquid/Sensors/Pressure & Temperature Sensor (TL)
      settings: SourceProductBaseCode=SS  InternalSimscapePortConfiguration="{\"Bottom\":[],\"Left\":[{\"id\":\"A\",\"label\":\"A\",\"type\":\"foundation.thermal_liquid.thermal_liquid\"}],\"Right\":[{\"id\":\"B\",\"label\":\"B\",\"type\":\"foundation.thermal_liquid.thermal_liquid\"},{\"id\":\"P\",\"label\":\"P\",\"type\":\"output\"},{\"id\":\"T\",\"label\":\"T\",\"type\":\"output\"}],\"Top\":[]}"
  Pump : Subsystem
  Cond O : PMIOPort  Side=Left
  Cond I : PMIOPort  Port=2  Side=Left
  Cab O : PMIOPort  Port=3  Side=Left
  Cab I : PMIOPort  Port=4  Side=Left
  Ref In : PMIOPort  Port=5  Side=Right
  Ref Out : PMIOPort  Port=6  Side=Right
  Bat I : PMIOPort  Port=7  Side=Right
  Bat O : PMIOPort  Port=8  Side=Right
  tag scope: T_lcc_out=global
  wires:
  PS-Simulink Converter/1 -> [T_lcc_out]
  connections:
  Ref Out/RConn1 -- LCC/RConn2
  Ref In/RConn1 -- LCC/RConn1
  Pump/LConn1 -- Cond I/RConn1 -- Cab I/RConn1 -- Bat I/RConn1
  Pump/RConn1 -- PTC Heater/LConn1 -- LCC/LConn1
  PS-Simulink Converter/LConn1 -- Pressure & Temperature Sensor (TL)/RConn3
  Absolute Reference (TL)/LConn1 -- Pressure & Temperature Sensor (TL)/RConn1
  Bat O/RConn1 -- Cab O/RConn1 -- Cond O/RConn1 -- Pressure & Temperature Sensor (TL)/LConn1 -- PTC Heater/RConn1 -- LCC/LConn2

== system Main_model/Motor + MC + GB (Front & Rear) ==
  Motor+MC+GB (Front+Rear) : Subsystem
      settings: PortSchema="{\"entries\":[{\"content\":{\"sides\":[{\"content\":{\"connectorIds\":[]},\"type\":\"ConnectorPlacement.EquallySpacedRectSide\",\"uuid\":\"56a66a49-7aa9-4955-aed7-55b7149df1a8\"},{\"content\":{\"connectorIds\":[],\"side\":\"RIGHT\"},\"type\":\"ConnectorPlacement.EquallySpacedRectSide\",\"uuid\":\"042c7100-8d59-436e-81e5-d4b9e3dba68e\"},{\"content\":{\"connectorIds\":[\"LConn1\",\"LConn2\"],\"side\":\"TOP\"},\"type\":\"ConnectorPlacement.EquallySpacedRectSide\",\"uuid\":\"dd4a5d99-9546-4656-ba80-8fb8ea1e7574\"}]},\"type\":\"ConnectorPlacement.EquallySpacedConnector\",\"uuid\":\"4ed40e14-40e7-49d7-8bc4-1dd0c573bf81\"}],\"packageUris\":[\"http://schema.mathworks.com/mf0/Connector/R2020b\"],\"version\":\"1.0\"}"
  Pump : Subsystem
  Bat O : PMIOPort  Side=Left
  Bat I : PMIOPort  Port=2  Side=Left
  Ch I : PMIOPort  Port=3  Side=Left
  Ch O : PMIOPort  Port=4  Side=Left
  Rad O : PMIOPort  Port=5  Side=Right
  Rad I : PMIOPort  Port=6  Side=Right
  connections:
  Rad I/RConn1 -- Pump/LConn1 -- Ch I/RConn1 -- Bat I/RConn1
  Ch O/RConn1 -- Motor+MC+GB (Front+Rear)/LConn1 -- Bat O/RConn1 -- Rad O/RConn1
  Motor+MC+GB (Front+Rear)/LConn2 -- Pump/RConn1

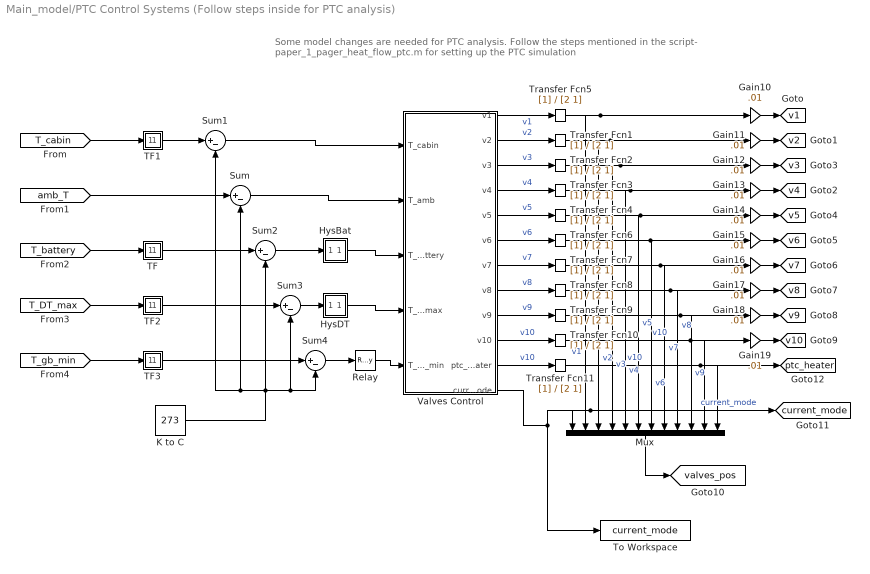
== system Main_model/PTC Control Systems (Follow steps inside for PTC analysis) ==
  note: Some model changes are needed for PTC analysis. Follow the steps mentioned in the script- paper_1_pager_heat_flow_ptc.m for setting up the PTC simulation
  Gain{10..19} (10 alike) : Gain  Gain=.01
  HysBat : Subsystem
  HysDT : Subsystem
  K to C : Constant  Value=273
  Mux : Mux  Inputs=12
  Relay : Relay  OnSwitchValue=T_DT_whr_active  OffSwitchValue=T_DT_whr_active-5  OnOutputValue=T_DT_whr_active*1.1  OffOutputValue=T_DT_whr_active*.9
  Sum{,1..4} (5 alike) : Sum  Inputs=|+-
  TF : Subsystem
  TF1 : Subsystem
  TF2 : Subsystem
  TF3 : Subsystem
  To Workspace : ToWorkspace  VariableName=current_mode  SaveFormat=Timeseries  SampleTime=-1
  Transfer Fcn{1..11} (11 alike) : TransferFcn  Denominator=[2 1]
  Valves Control : MATLAB Function  TreatAsAtomicUnit=on
  tag scope: current_mode=global, ptc_heater=global, v10=global, v1=global, v2=global, v3=global, v4=global, v5=global, v6=global, v7=global, v8=global, v9=global, valves_pos=global
  wires:
  Sum3/1 -> HysDT/1(In1)
  Transfer Fcn7/1 -> Gain16/1, Mux/8  "v7"
  [amb_T] -> Sum/1
  Mux/1 -> [valves_pos]
  Valves Control/1(v1) -> Transfer Fcn5/1  "v1"
  Gain15/1 -> [v6]
  Transfer Fcn5/1 -> Gain10/1, Mux/2  "v1"
  Valves Control/8(v8) -> Transfer Fcn8/1  "v8"
  Valves Control/7(v7) -> Transfer Fcn7/1  "v7"
  Sum1/1 -> Valves Control/1(T_cabin)
  Transfer Fcn4/1 -> Gain14/1, Mux/6  "v5"
  Gain13/1 -> [v4]
  Valves Control/12(current_mode) -> [current_mode], Mux/1, To Workspace/1  "current_mode"
  Gain17/1 -> [v8]
  HysBat/1(Out1) -> Valves Control/3(T_battery)
  Gain16/1 -> [v7]
  Valves Control/9(v9) -> Transfer Fcn9/1  "v9"
  Gain14/1 -> [v5]
  Gain12/1 -> [v3]
  Transfer Fcn1/1 -> Gain11/1, Mux/3  "v2"
  Gain19/1 -> [v10]
  Sum4/1 -> Relay/1
  Transfer Fcn9/1 -> Gain18/1, Mux/10  "v9"
  Gain11/1 -> [v2]
  Transfer Fcn2/1 -> Gain12/1, Mux/4  "v3"
  Valves Control/3(v3) -> Transfer Fcn2/1  "v3"
  Transfer Fcn8/1 -> Gain17/1, Mux/9  "v8"
  Gain10/1 -> [v1]
  Transfer Fcn6/1 -> Gain15/1, Mux/7  "v6"
  Transfer Fcn10/1 -> Gain19/1, Mux/11  "v10"
  Transfer Fcn3/1 -> Gain13/1, Mux/5  "v4"
  Valves Control/6(v6) -> Transfer Fcn6/1  "v6"
  Gain18/1 -> [v9]
  Valves Control/4(v4) -> Transfer Fcn3/1  "v4"
  Valves Control/10(v10) -> Transfer Fcn10/1  "v10"
  Valves Control/5(v5) -> Transfer Fcn4/1  "v5"
  Sum/1 -> Valves Control/2(T_amb)
  Sum2/1 -> HysBat/1(In1)
  K to C/1 -> Sum4/2, Sum3/2, Sum2/2, Sum/2, Sum1/2
  Valves Control/2(v2) -> Transfer Fcn1/1  "v2"
  [T_gb_min] -> TF3/1(In1)
  [T_battery] -> TF/1(In1)
  [T_cabin] -> TF1/1(In1)
  [T_DT_max] -> TF2/1(In1)
  TF1/1(Out1) -> Sum1/1
  TF3/1(Out1) -> Sum4/1
  TF2/1(Out1) -> Sum3/1
  TF/1(Out1) -> Sum2/1
  HysDT/1(Out1) -> Valves Control/4(T_DT_max)
  Relay/1 -> Valves Control/5(T_DT_min)
  Valves Control/11(ptc_heater) -> Transfer Fcn11/1  "v10"
  Transfer Fcn11/1 -> [ptc_heater], Mux/12  "v10"

== system Main_model/Radiator ==
  Pump : Subsystem
  Thermal Liquid Properties (TL) : SimscapeFluids_lib/Thermal Liquid/Utilities/Thermal Liquid Properties (TL)  fluid_list=fluids.thermal_liquid.utilities.enum.thermal_liquid_fluid_list.ethylene_glycol  concentration_param_EG=fluids.thermal_liquid.utilities.enum.thermal_liquid_concentration.volume_fraction  concentration_param_PG=fluids.thermal_liquid.utilities.enum.thermal_liquid_concentration.volume_fraction  c_mass_SW=3.5e-3  c_mass_EG=.4  c_mass_PG=0.1  c_mass_GL=0.1  c_vol_EG=coolant_ethylene_glycol_vol_frac  c_vol_PG=0.1  beta_const_EG=2.1791 GPa  beta_const_PG=2.1791 GPa  beta_const_GL=2.1791 GPa  p_min_EG=0.01 MPa  p_min_PG=0.01 MPa  p_min_GL=0.01 MPa  p_max_EG=50 MPa  p_max_PG=50 MPa  p_max_GL=50 MPa  p_atm=ambient_pressure MPa
      settings: SourceProductBaseCode=SH
  radiator : Subsystem
      settings: PortSchema="{\"entries\":[{\"content\":{\"sides\":[{\"content\":{\"connectorIds\":[]},\"type\":\"ConnectorPlacement.EquallySpacedRectSide\",\"uuid\":\"3be5e3bd-c423-4591-b0f7-380c1ba81e55\"},{\"content\":{\"connectorIds\":[],\"side\":\"RIGHT\"},\"type\":\"ConnectorPlacement.EquallySpacedRectSide\",\"uuid\":\"149d4538-0447-4c3c-bea8-6305fc9625c0\"},{\"content\":{\"connectorIds\":[\"LConn1\",\"LConn2\"],\"side\":\"TOP\"},\"type\":\"ConnectorPlacement.EquallySpacedRectSide\",\"uuid\":\"dd60c3f6-9393-4002-a01b-9d7c883b77f2\"}]},\"type\":\"ConnectorPlacement.EquallySpacedConnector\",\"uuid\":\"8455fa94-fdd0-4f54-8085-fe1f60725002\"}],\"packageUris\":[\"http://schema.mathworks.com/mf0/Connector/R2020b\"],\"version\":\"1.0\"}"
  Bat I : PMIOPort  Side=Right
  Bat O : PMIOPort  Port=2  Side=Right
  DT I : PMIOPort  Port=3  Side=Right
  DT O : PMIOPort  Port=4  Side=Right
  connections:
  radiator/LConn2 -- Bat O/RConn1 -- Thermal Liquid Properties (TL)/RConn1 -- DT O/RConn1
  Bat I/RConn1 -- Pump/LConn1 -- DT I/RConn1
  radiator/LConn1 -- Pump/RConn1

== system Main_model/TXV ==
  Cap (2P) : fl_lib/Two-Phase Fluid/Elements/Cap (2P)  p_specify=off  p_priority=None  p=0.101325 MPa  p_nominal_specify=off  p_nominal_unit=MPa  p_nominal_value=1  u_specify=off  u_priority=None  u=1.5e+3 kJ/kg  u_nominal_specify=off  u_nominal_unit=kJ/kg  u_nominal_value=1
      settings: SourceProductBaseCode=SS  InternalSimscapePortConfiguration="{\"Bottom\":[],\"Left\":[{\"id\":\"A\",\"label\":\"\",\"type\":\"foundation.two_phase_fluid.two_phase_fluid\"}],\"Right\":[],\"Top\":[]}"
  Cap (2P)1 : fl_lib/Two-Phase Fluid/Elements/Cap (2P)  p_specify=off  p_priority=None  p=0.101325 MPa  p_nominal_specify=off  p_nominal_unit=MPa  p_nominal_value=1  u_specify=off  u_priority=None  u=1.5e+3 kJ/kg  u_nominal_specify=off  u_nominal_unit=kJ/kg  u_nominal_value=1
      settings: SourceProductBaseCode=SS  InternalSimscapePortConfiguration="{\"Bottom\":[],\"Left\":[{\"id\":\"A\",\"label\":\"\",\"type\":\"foundation.two_phase_fluid.two_phase_fluid\"}],\"Right\":[],\"Top\":[]}"
  Conductive Heat Transfer : fl_lib/Thermal/Thermal Elements/Conductive Heat Transfer  Commented=on  area=pi*ref_pipe_dia*0.02 m^2  thickness=ref_pipe_thickness m  th_cond=al_conductivity W/(m*K)  T_specify=off  T_priority=None  T=0 K  T_nominal_specify=off  T_nominal_unit=K  T_nominal_value=1  Q_specify=off  Q_priority=None  Q=0 W  Q_nominal_specify=off  Q_nominal_unit=W  Q_nominal_value=1
  Expansion Valve : SimscapeFluids_lib/Two-Phase Fluid/Valves & Orifices/Flow Control Valves/Thermostatic Expansion Valve (2P)  Q_nominal=2*txv_nom_capacity W  Q_max=2*txv_max_capacity W  T_evap=evap_nom_temp K  delta_T_static=evap_min_superheat_delta deltaK  delta_T_nominal=evap_nom_superheat_delta deltaK  T_cond=cond_nom_temp K  delta_T_sub=cond_nom_subcool_delta deltaK  pressure_equalization=fluids.two_phase_fluid.valves_orifices.flow_control_valves.enum.ThermostaticExpansionValveEqualization.External  mop=fluids.two_phase_fluid.valves_orifices.flow_control_valves.enum.ThermostaticExpansionValveMOP.Off  p_mop=.8 MPa  T_mop=288.15 K  bulb_dynamics=simscape.enum.onoff.off  tau_bulb=0.1 s  area=refrigerant_pipe_cross_sec_area m^2  mdot_leak_fraction=1e-6  smoothing_factor=0.01  B_lam=0.999  tau_x=0.1 s
      settings: SourceProductBaseCode=SH  InternalSimscapePortConfiguration="{\"Bottom\":[],\"Left\":[{\"id\":\"A\",\"label\":\"A\",\"type\":\"foundation.two_phase_fluid.two_phase_fluid\"}],\"Right\":[{\"id\":\"B\",\"label\":\"B\",\"type\":\"foundation.two_phase_fluid.two_phase_fluid\"}],\"Top\":[{\"id\":\"S\",\"label\":\"S\",\"type\":\"foundation.two_phase_fluid.two_phase_fluid\"},{\"id\":\"E\",\"label\":\"E\",\"type\":\"foundation.two_phase_fluid.two_phase_fluid\"}]}"
  Perfect Insulator : fl_lib/Thermal/Thermal Elements/Perfect Insulator  T_specify=off  T_priority=None  T=0 K  T_nominal_specify=off  T_nominal_unit=K  T_nominal_value=1
  Receiver : SimscapeFluids_lib/Two-Phase Fluid/Tanks & Accumulators/Receiver Accumulator (2P)  volume=refrigerant_tank_vol l  area_AV=0.01 m^2  area_BV=0.01 m^2  area_AL=refrigerant_pipe_cross_sec_area m^2  area_BL=refrigerant_pipe_cross_sec_area m^2  V_frac_error=simscape.enum.assert.action.none  V_frac_min=0.05  V_frac_max=0.95  V_frac_smooth=0.05  p_crit_error=simscape.enum.assert.action.warn  hc_vap=20 W/(m^2*K)  hc_liq=100 W/(m^2*K)  surface_area=0.1 m^2  receiver_accumulator_energy_spec=fluids.two_phase_fluid.enum.receiver_accumulator_energy_spec.volume_fraction  p_init=refrigerant_initial_P MPa  T_init=refrigerant_initial_T K  M_frac_init=0.5  V_frac_init=1-refrigerant_initial_void_fraction  h_init=1500 kJ/kg  u_init=1500 kJ/kg  tau_vap_cond=1 s
      settings: SourceProductBaseCode=SH  InternalSimscapePortConfiguration="{\"Bottom\":[],\"Left\":[{\"id\":\"AV\",\"label\":\"AV\",\"type\":\"foundation.two_phase_fluid.two_phase_fluid\"},{\"id\":\"AL\",\"label\":\"AL\",\"type\":\"foundation.two_phase_fluid.two_phase_fluid\"},{\"id\":\"H\",\"label\":\"H\",\"type\":\"foundation.thermal.thermal\"}],\"Right\":[{\"id\":\"BV\",\"label\":\"BV\",\"type\":\"foundation.two_phase_fluid.two_phase_fluid\"},{\"id\":\"BL\",\"label\":\"BL\",\"type\":\"foundation.two_phase_fluid.two_phase_fluid\"},{\"id\":\"L\",\"label\":\"L\",\"type\":\"output\"}],\"Top\":[]}"
  Solver Configuration : nesl_utility/Solver Configuration  PhysicalDomain=network_engine_domain  SubClassName=solver  LeftPortType=input  RightPortType=generic  Tones=[]  Harmonics=[]  SimulateNoise=off  Profile=off  UseLocalSampling=off  EnableSwitchedLinearOptims=on  FrequencyDomain=off  UseCCode=off  RelTol=0.001  AbsTol=1e-06  MinStep=1e-09  ToWorkspace=off  RevertToSquareIcSolve=off  NumHomotopyIterations=100  PhasorMode=off  PhasorModeNumHarmonics=1  DoDC=off  ResidualTolerance=1e-09  UseLocalSolver=off  LocalSolverChoice=NE_BACKWARD_EULER_ADVANCER  LocalSolverSampleTime=0.001  DoFixedCost=off  MaxNonlinIter=3  MaxModeIter=2  ComputeImpulses=off  ImpulseIterations=2  LinearAlgebra=auto  EquationFormulation=NE_TIME_EF  DelaysMemoryBudget=1024  AutomaticFiltering=on  FilteringTimeConstant=0.001  PartitionStorageMethod=AS_NEEDED  PartitionMemoryBudget=1024  PartitionMethod=ROBUST
      settings: SourceProductBaseCode=PW,SS
  Thermal Mass : fl_lib/Thermal/Thermal Elements/Thermal Mass  Commented=on  mass=.05 kg  sp_heat=447 J/(K*kg)  T_specify=off  T_priority=High  T=300 K  T_nominal_specify=off  T_nominal_unit=K  T_nominal_value=1  Q_specify=off  Q_priority=None  Q=0 W  Q_nominal_specify=off  Q_nominal_unit=W  Q_nominal_value=1
  Thermostatic Expansion Valve (2P) : SimscapeFluids_lib/Two-Phase Fluid/Valves & Orifices/Flow Control Valves/Thermostatic Expansion Valve (2P)  Q_nominal=15 kW  Q_max=20 kW  T_evap=278.15 K  delta_T_static=5 deltaK  delta_T_nominal=10 deltaK  T_cond=313.15 K  delta_T_sub=5 deltaK  pressure_equalization=fluids.two_phase_fluid.valves_orifices.flow_control_valves.enum.ThermostaticExpansionValveEqualization.Internal  mop=fluids.two_phase_fluid.valves_orifices.flow_control_valves.enum.ThermostaticExpansionValveMOP.Off  p_mop=0.5 MPa  T_mop=288.15 K  bulb_dynamics=simscape.enum.onoff.off  tau_bulb=20 s  area=0.01 m^2  mdot_leak_fraction=1e-6  smoothing_factor=0.01  B_lam=0.999  tau_x=0.1 s
      settings: SourceProductBaseCode=SH  InternalSimscapePortConfiguration="{\"Bottom\":[],\"Left\":[{\"id\":\"A\",\"label\":\"A\",\"type\":\"foundation.two_phase_fluid.two_phase_fluid\"}],\"Right\":[{\"id\":\"B\",\"label\":\"B\",\"type\":\"foundation.two_phase_fluid.two_phase_fluid\"}],\"Top\":[{\"id\":\"S\",\"label\":\"S\",\"type\":\"foundation.two_phase_fluid.two_phase_fluid\"}]}"
  heat loss : Subsystem
  "Bulb " : PMIOPort  Side=Left
  Ref Out : PMIOPort  Port=2  Side=Left
  Ref In : PMIOPort  Port=3  Side=Right
  connections:
  "Bulb "/RConn1 -- Expansion Valve/LConn2 -- Expansion Valve/LConn3
  Perfect Insulator/LConn1 -- Receiver/LConn3
  Cap (2P)1/LConn1 -- Receiver/RConn1
  Cap (2P)/LConn1 -- Receiver/LConn1
  Expansion Valve/LConn1 -- Receiver/RConn2
  heat loss/RConn1 -- Ref Out/RConn1
  Solver Configuration/RConn1 -- Ref In/RConn1 -- Receiver/LConn2
  heat loss/LConn1 -- Expansion Valve/RConn1

== system Main_model/v10a ==
  Gate Valve (TL) : SimscapeFluids_lib/Thermal Liquid/Valves & Orifices/Flow Control Valves/Gate Valve (TL)  diam_orifice=valve_orifice_dia m  x_0=0 m  area_leak=valve_leakage_area m^2  smoothing_factor=valve_smoothing_factor  area=valve_cross_sec_area m^2  length=0.1 m  Cd=0.7  Re_c=12
      settings: SourceProductBaseCode=SH  InternalSimscapePortConfiguration="{\"Bottom\":[],\"Left\":[{\"id\":\"A\",\"label\":\"A\",\"type\":\"foundation.thermal_liquid.thermal_liquid\"},{\"id\":\"S\",\"label\":\"S\",\"type\":\"input\"}],\"Right\":[{\"id\":\"B\",\"label\":\"B\",\"type\":\"foundation.thermal_liquid.thermal_liquid\"}],\"Top\":[]}"
  Simulink-PS Converter1 : nesl_utility/Simulink-PS Converter  PhysicalDomain=network_engine_domain  SubClassName=ps_input  LeftPortType=input  RightPortType=output  PseudoPeriodic=off  Frequencies=[]  NoiseDistribution=none  NoiseParameters=[]  Unit=1  AffineConversion=off  FilteringAndDerivatives=provide  SimscapeFilterOrder=1  InputFilterTimeConstant=0.001  UdotUserProvided=0
      settings: SourceProductBaseCode=PW,SS
  Switch : Switch  Criteria=u2 > Threshold
  1 : PMIOPort  Side=Left
  2 : PMIOPort  Port=2  Side=Right
  wires:
  [v10a] -> Switch/1
  [v10] -> Switch/3
  [switch] -> Switch/2
  Switch/1 -> Simulink-PS Converter1/1
  connections:
  Gate Valve (TL)/RConn1 -- 2/RConn1
  Gate Valve (TL)/LConn2 -- Simulink-PS Converter1/RConn1
  Gate Valve (TL)/LConn1 -- 1/RConn1
